simulink library "aero_libdap"  (Simulink 6.0)
settings: Solver=ode45  SolverMode=SingleTasking  StartTime=0.0  StopTime=10.0  RelTol=1e-3
values from neighbouring files (symbols this model uses):
  DB = u(6)    [aero_phaseplane.m]
  delt = 0.1    [aero_pointer_tracker.m]
undefined symbols (not defined in the file or in its folder): tmin
settings Model: CovMetricSettings=d  Creator=The MathWorks Inc.  LastModifiedBy=batserve  ExtModeAutoUpdateStatusClock=off
settings OptimizationCC: BooleanDataType=off
settings DebuggingCC: CheckExecutionContextPreStartOutputMsg=on  CheckExecutionContextRuntimeOutputMsg=on  SolverPrmCheckMsg=none
settings HardwareCC: TargetUnknown=on

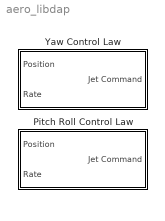
== system aero_libdap ==
  Pitch Roll Control Law : Subsystem  PropExecContextAcrossSSBoundary=on  mask(Control Law){alph=, alphs=, DB=DB, tmin=tmin, delt=delt}
      mask prompts: alph "Single Jet Accel:"; alphs "Single Jet Switch Curve Accel:"; DB "Dead Band:"; tmin "Min. Jet On Time:"; delt "Sample Time:"
      mask help: Implements Control Law for the LM. Works for yaw, u and v jet axes.
  Yaw Control Law : Subsystem  PropExecContextAcrossSSBoundary=on  mask(Control Law){alph=, alphs=, DB=DB, tmin=tmin, delt=delt}
      mask prompts: alph "Single Jet Accel:"; alphs "Single Jet Switch Curve Accel:"; DB "Dead Band:"; tmin "Min Jet On Time:"; delt "Sample Time:"
      mask help: Implements Control Law for the LM. Works for yaw, u and v jet axes.

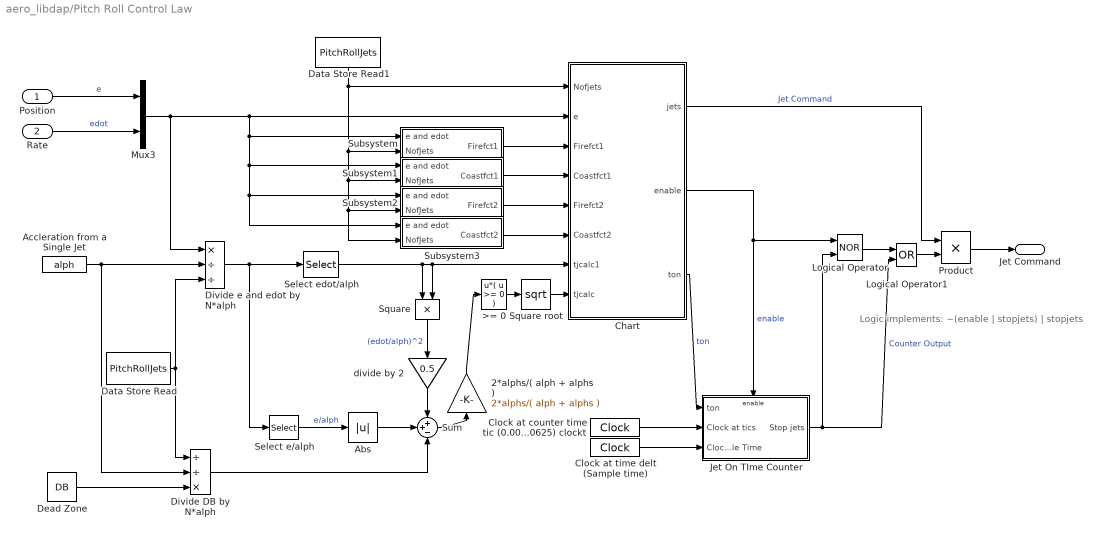
== system aero_libdap/Pitch Roll Control Law ==
  note: Logic implements:
      | ~(enable | stopjets) | stopjets
  Position : Inport  Port=1  LatchInput=off
  Rate : Inport  Port=2  LatchInput=off
  2*alphs/( alph + alphs ) : Gain  Orientation=up  Gain=2*alphs/( alph + alphs )  SaturateOnIntegerOverflow=on
  >= 0 : Fcn  Expr=u*( u >= 0 )
  Abs : Abs  SaturateOnIntegerOverflow=on
  Accleration from a Single Jet : Constant  Value=alph
  Chart : Stateflow chart  PropExecContextAcrossSSBoundary=on
  Clock at counter time tic (0.000625) clockt : DigitalClock  SampleTime=0.000625
  Clock at time delt (Sample time) : DigitalClock  SampleTime=delt
  Data Store Read : DataStoreRead  DialogController=Simulink.DDGSource  DataStoreName=PitchRollJets  SampleTime=delt
  Data Store Read1 : DataStoreRead  Orientation=down  DialogController=Simulink.DDGSource  DataStoreName=PitchRollJets  SampleTime=delt
  Dead Zone : Constant  Value=DB
  Divide e and edot by N*alph : Product  Inputs=*//  SaturateOnIntegerOverflow=on  RndMeth=Zero  InputSameDT=on
  Divide DB by N*alph : Product  Inputs=//*  SaturateOnIntegerOverflow=on  RndMeth=Zero  InputSameDT=on
  Jet On TIme Counter : Subsystem  TreatAsAtomicUnit=on  PropExecContextAcrossSSBoundary=on
  Logical Operator : Logic  Operator=NOR
  Logical Operator1 : Logic  Operator=OR
  Mux3 : Mux  Inputs=2
  Product : Product  SaturateOnIntegerOverflow=on  RndMeth=Zero  InputSameDT=on
  Select e/alph : Selector  Elements=[1]  InputPortWidth=2
  Select edot/alph : Selector  Elements=[2]  InputPortWidth=2
  Square : Product  Orientation=down  SaturateOnIntegerOverflow=on  RndMeth=Zero  InputSameDT=on
  Square root : Math  Operator=sqrt  SaturateOnIntegerOverflow=on
  Subsystem : Subsystem  PropExecContextAcrossSSBoundary=on
  Subsystem1 : Subsystem  PropExecContextAcrossSSBoundary=on
  Subsystem2 : Subsystem  PropExecContextAcrossSSBoundary=on
  Subsystem3 : Subsystem  PropExecContextAcrossSSBoundary=on
  Sum : Sum  Inputs=++-  SaturateOnIntegerOverflow=on  InputSameDT=on
  divide by 2 : Gain  Orientation=down  Gain=0.5  SaturateOnIntegerOverflow=on
  Jet Command : Outport  InitialOutput=0
  wires:
  Data Store Read1/1 -> Subsystem3/2(NofJets), Subsystem2/2(NofJets), Subsystem1/2(NofJets), Subsystem/2(NofJets), Chart/1(Nofjets)
  Rate/1 -> Mux3/2  "edot"
  Position/1 -> Mux3/1  "e"
  Mux3/1 -> Chart/2(e), Divide e and edot by N*alph/1, Subsystem/1(e and edot), Subsystem1/1(e and edot), Subsystem2/1(e and edot), Subsystem3/1(e and edot)
  Square/1 -> divide by 2/1  "(edot/alph)^2"
  Square root/1 -> Chart/8(tjcalc)
  Chart/1(jets) -> Product/1  "Jet Command"
  Select edot/alph/1 -> Square/1, Chart/7(tjcalc1), Square/2
  Select e/alph/1 -> Abs/1  "e/alph"
  divide by 2/1 -> Sum/1
  Sum/1 -> 2*alphs/( alph + alphs )/1
  Abs/1 -> Sum/2
  Divide e and edot by N*alph/1 -> Select edot/alph/1, Select e/alph/1
  Data Store Read/1 -> Divide e and edot by N*alph/3, Divide DB by N*alph/1
  Accleration from a Single Jet/1 -> Divide e and edot by N*alph/2, Divide DB by N*alph/2
  Dead Zone/1 -> Divide DB by N*alph/3
  Divide DB by N*alph/1 -> Sum/3
  Chart/2(enable) -> Jet On TIme Counter/Enable, Logical Operator/1  "enable"
  Logical Operator1/1 -> Product/2
  Chart/3(ton) -> Jet On TIme Counter/1(ton)  "ton"
  Clock at counter time tic (0.000625) clockt/1 -> Jet On TIme Counter/2(Clock at tics)
  Clock at time delt (Sample time)/1 -> Jet On TIme Counter/3(Clock at Sample Time)
  Jet On TIme Counter/1(Stop jets) -> Logical Operator/2, Logical Operator1/2  "Counter Output"
  Logical Operator/1 -> Logical Operator1/1
  Subsystem3/1(Coastfct2) -> Chart/6(Coastfct2)
  Subsystem2/1(Firefct2) -> Chart/5(Firefct2)
  Subsystem1/1(Coastfct1) -> Chart/4(Coastfct1)
  Subsystem/1(Firefct1) -> Chart/3(Firefct1)
  Product/1 -> Jet Command/1
  2*alphs/( alph + alphs )/1 -> >= 0/1
  >= 0/1 -> Square root/1

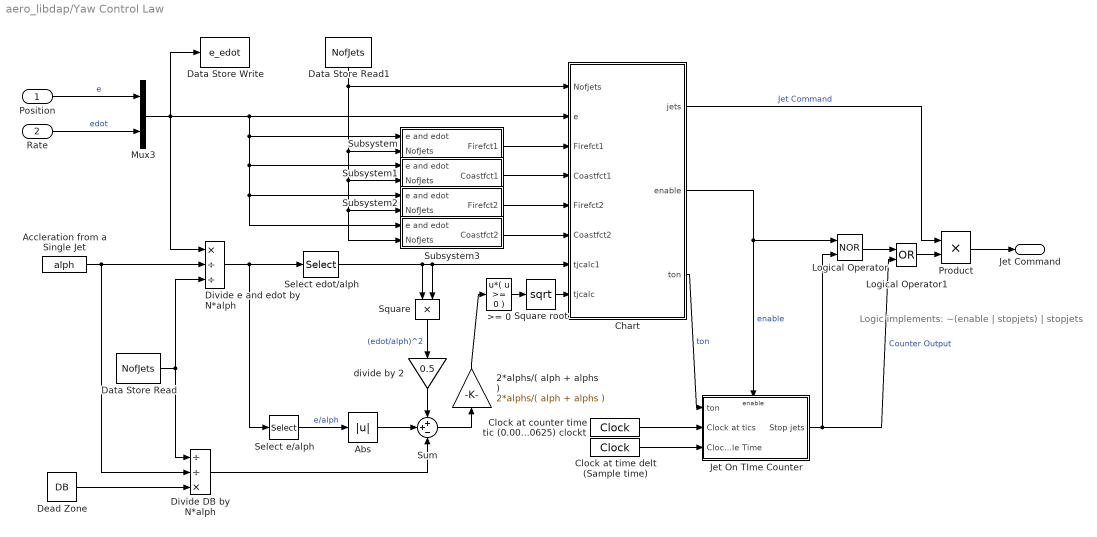
== system aero_libdap/Yaw Control Law ==
  note: Logic implements:
      | ~(enable | stopjets) | stopjets
  Position : Inport  Port=1  LatchInput=off
  Rate : Inport  Port=2  LatchInput=off
  2*alphs/( alph + alphs ) : Gain  Orientation=up  Gain=2*alphs/( alph + alphs )  SaturateOnIntegerOverflow=on
  >= 0 : Fcn  Expr=u*( u >= 0 )
  Abs : Abs  SaturateOnIntegerOverflow=on
  Accleration from a Single Jet : Constant  Value=alph
  Chart : Stateflow chart  PropExecContextAcrossSSBoundary=on
  Clock at counter time tic (0.000625) clockt : DigitalClock  SampleTime=0.000625
  Clock at time delt (Sample time) : DigitalClock  SampleTime=delt
  Data Store Read : DataStoreRead  DialogController=Simulink.DDGSource  DataStoreName=NofJets  SampleTime=delt
  Data Store Read1 : DataStoreRead  Orientation=down  DialogController=Simulink.DDGSource  DataStoreName=NofJets  SampleTime=delt
  Data Store Write : DataStoreWrite  DialogController=Simulink.DDGSource  DataStoreName=e_edot  SampleTime=-1
  Dead Zone : Constant  Value=DB
  Divide e and edot by N*alph : Product  Inputs=*//  SaturateOnIntegerOverflow=on  RndMeth=Zero  InputSameDT=on
  Divide DB by N*alph : Product  Inputs=//*  SaturateOnIntegerOverflow=on  RndMeth=Zero  InputSameDT=on
  Jet On TIme Counter : Subsystem  TreatAsAtomicUnit=on  PropExecContextAcrossSSBoundary=on
  Logical Operator : Logic  Operator=NOR
  Logical Operator1 : Logic  Operator=OR
  Mux3 : Mux  Inputs=2
  Product : Product  SaturateOnIntegerOverflow=on  RndMeth=Zero  InputSameDT=on
  Select e/alph : Selector  Elements=[1]  InputPortWidth=2
  Select edot/alph : Selector  Elements=[2]  InputPortWidth=2
  Square : Product  Orientation=down  SaturateOnIntegerOverflow=on  RndMeth=Zero  InputSameDT=on
  Square root : Math  Operator=sqrt  SaturateOnIntegerOverflow=on
  Subsystem : Subsystem  PropExecContextAcrossSSBoundary=on
  Subsystem1 : Subsystem  PropExecContextAcrossSSBoundary=on
  Subsystem2 : Subsystem  PropExecContextAcrossSSBoundary=on
  Subsystem3 : Subsystem  PropExecContextAcrossSSBoundary=on
  Sum : Sum  Inputs=++-  SaturateOnIntegerOverflow=on  InputSameDT=on
  divide by 2 : Gain  Orientation=down  Gain=0.5  SaturateOnIntegerOverflow=on
  Jet Command : Outport  InitialOutput=0
  wires:
  Product/1 -> Jet Command/1
  Subsystem/1(Firefct1) -> Chart/3(Firefct1)
  Subsystem1/1(Coastfct1) -> Chart/4(Coastfct1)
  Subsystem2/1(Firefct2) -> Chart/5(Firefct2)
  Subsystem3/1(Coastfct2) -> Chart/6(Coastfct2)
  Logical Operator/1 -> Logical Operator1/1
  Jet On TIme Counter/1(Stop jets) -> Logical Operator1/2, Logical Operator/2  "Counter Output"
  Clock at time delt (Sample time)/1 -> Jet On TIme Counter/3(Clock at Sample Time)
  Clock at counter time tic (0.000625) clockt/1 -> Jet On TIme Counter/2(Clock at tics)
  Chart/3(ton) -> Jet On TIme Counter/1(ton)  "ton"
  Logical Operator1/1 -> Product/2
  Chart/2(enable) -> Logical Operator/1, Jet On TIme Counter/Enable  "enable"
  Divide DB by N*alph/1 -> Sum/3
  Dead Zone/1 -> Divide DB by N*alph/3
  Accleration from a Single Jet/1 -> Divide DB by N*alph/2, Divide e and edot by N*alph/2
  Data Store Read/1 -> Divide DB by N*alph/1, Divide e and edot by N*alph/3
  Divide e and edot by N*alph/1 -> Select e/alph/1, Select edot/alph/1
  Abs/1 -> Sum/2
  Sum/1 -> 2*alphs/( alph + alphs )/1
  divide by 2/1 -> Sum/1
  Select e/alph/1 -> Abs/1  "e/alph"
  Select edot/alph/1 -> Square/2, Chart/7(tjcalc1), Square/1
  Chart/1(jets) -> Product/1  "Jet Command"
  Square root/1 -> Chart/8(tjcalc)
  Square/1 -> divide by 2/1  "(edot/alph)^2"
  Mux3/1 -> Subsystem3/1(e and edot), Subsystem2/1(e and edot), Subsystem1/1(e and edot), Subsystem/1(e and edot), Divide e and edot by N*alph/1, Chart/2(e), Data Store Write/1
  Position/1 -> Mux3/1  "e"
  Rate/1 -> Mux3/2  "edot"
  Data Store Read1/1 -> Chart/1(Nofjets), Subsystem/2(NofJets), Subsystem1/2(NofJets), Subsystem2/2(NofJets), Subsystem3/2(NofJets)
  2*alphs/( alph + alphs )/1 -> >= 0/1
  >= 0/1 -> Square root/1

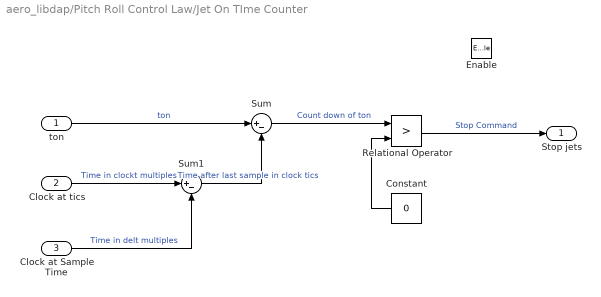
== system aero_libdap/Pitch Roll Control Law/Jet On TIme Counter ==
  ton : Inport  Port=1  LatchInput=off
  Clock at tics : Inport  Port=2  LatchInput=off
  Clock at Sample Time : Inport  Port=3  LatchInput=off
  Enable : EnablePort  StatesWhenEnabling=reset
  Constant : Constant  Orientation=left  Value=0
  Relational Operator : RelationalOperator  Operator=>  InputSameDT=on
  Sum : Sum  Inputs=|+-  SaturateOnIntegerOverflow=on  InputSameDT=on
  Sum1 : Sum  Inputs=|+-  SaturateOnIntegerOverflow=on  InputSameDT=on
  Stop jets : Outport
  wires:
  Constant/1 -> Relational Operator/2
  ton/1 -> Sum/1  "ton"
  Clock at tics/1 -> Sum1/1  "Time in clockt multiples"
  Clock at Sample Time/1 -> Sum1/2  "Time in delt multiples"
  Sum1/1 -> Sum/2  "Time after last sample in clock tics"
  Sum/1 -> Relational Operator/1  "Count down of ton"
  Relational Operator/1 -> Stop jets/1  "Stop Command"

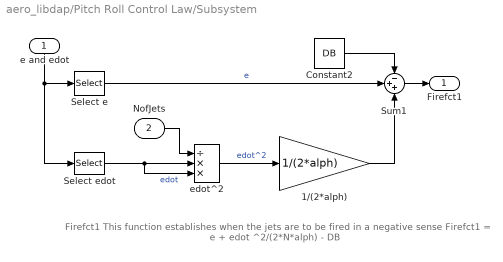
== system aero_libdap/Pitch Roll Control Law/Subsystem ==
  note: Firefct1
      | This function establishes when the jets are to be fired in a negative sense
      | Firefct1 = e + edot ^2/(2*N*alph) - DB
  e and edot : Inport  Orientation=down  Port=1  LatchInput=off
  NofJets : Inport  Port=2  LatchInput=off
  1/(2*alph) : Gain  Gain=1/(2*alph)  SaturateOnIntegerOverflow=on
  Constant2 : Constant  Value=DB
  Select e : Selector  Elements=[1]  InputPortWidth=2
  Select edot : Selector  Elements=[2]  InputPortWidth=2
  Sum1 : Sum  Inputs=-++  SaturateOnIntegerOverflow=on  InputSameDT=on
  edot^2 : Product  Inputs=/**  SaturateOnIntegerOverflow=on  RndMeth=Zero  InputSameDT=on
  Firefct1 : Outport
  wires:
  edot^2/1 -> 1/(2*alph)/1  "edot^2"
  Select edot/1 -> edot^2/2, edot^2/3  "edot"
  NofJets/1 -> edot^2/1
  e and edot/1 -> Select e/1, Select edot/1
  1/(2*alph)/1 -> Sum1/3
  Constant2/1 -> Sum1/1
  Select e/1 -> Sum1/2  "e"
  Sum1/1 -> Firefct1/1

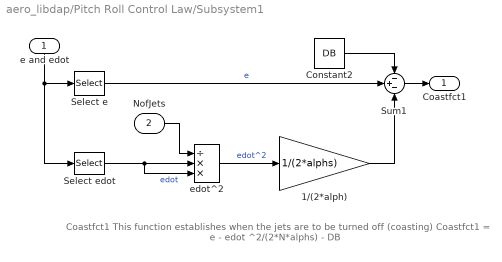
== system aero_libdap/Pitch Roll Control Law/Subsystem1 ==
  note: Coastfct1
      | This function establishes when the jets are to be turned off (coasting)
      | Coastfct1 = e - edot ^2/(2*N*alphs) - DB
  e and edot : Inport  Orientation=down  Port=1  LatchInput=off
  NofJets : Inport  Port=2  LatchInput=off
  1/(2*alph) : Gain  Gain=1/(2*alphs)  SaturateOnIntegerOverflow=on
  Constant2 : Constant  Value=DB
  Select e : Selector  Elements=[1]  InputPortWidth=2
  Select edot : Selector  Elements=[2]  InputPortWidth=2
  Sum1 : Sum  Inputs=-+-  SaturateOnIntegerOverflow=on  InputSameDT=on
  edot^2 : Product  Inputs=/**  SaturateOnIntegerOverflow=on  RndMeth=Zero  InputSameDT=on
  Coastfct1 : Outport
  wires:
  Sum1/1 -> Coastfct1/1
  Select e/1 -> Sum1/2  "e"
  Constant2/1 -> Sum1/1
  1/(2*alph)/1 -> Sum1/3
  e and edot/1 -> Select edot/1, Select e/1
  NofJets/1 -> edot^2/1
  Select edot/1 -> edot^2/3, edot^2/2  "edot"
  edot^2/1 -> 1/(2*alph)/1  "edot^2"

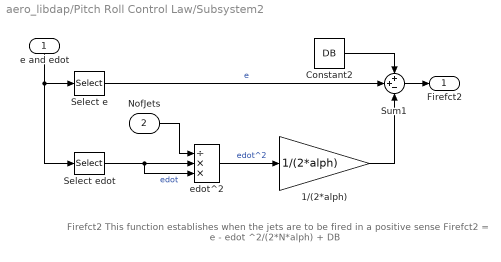
== system aero_libdap/Pitch Roll Control Law/Subsystem2 ==
  note: Firefct2
      | This function establishes when the jets are to be fired in a positive sense
      | Firefct2 = e - edot ^2/(2*N*alph) + DB
  e and edot : Inport  Orientation=down  Port=1  LatchInput=off
  NofJets : Inport  Port=2  LatchInput=off
  1/(2*alph) : Gain  Gain=1/(2*alph)  SaturateOnIntegerOverflow=on
  Constant2 : Constant  Value=DB
  Select e : Selector  Elements=[1]  InputPortWidth=2
  Select edot : Selector  Elements=[2]  InputPortWidth=2
  Sum1 : Sum  Inputs=++-  SaturateOnIntegerOverflow=on  InputSameDT=on
  edot^2 : Product  Inputs=/**  SaturateOnIntegerOverflow=on  RndMeth=Zero  InputSameDT=on
  Firefct2 : Outport
  wires:
  edot^2/1 -> 1/(2*alph)/1  "edot^2"
  Select edot/1 -> edot^2/2, edot^2/3  "edot"
  NofJets/1 -> edot^2/1
  e and edot/1 -> Select e/1, Select edot/1
  1/(2*alph)/1 -> Sum1/3
  Constant2/1 -> Sum1/1
  Select e/1 -> Sum1/2  "e"
  Sum1/1 -> Firefct2/1

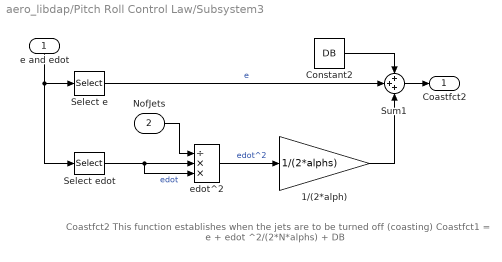
== system aero_libdap/Pitch Roll Control Law/Subsystem3 ==
  note: Coastfct2
      | This function establishes when the jets are to be turned off (coasting)
      | Coastfct1 = e + edot ^2/(2*N*alphs) + DB
  e and edot : Inport  Orientation=down  Port=1  LatchInput=off
  NofJets : Inport  Port=2  LatchInput=off
  1/(2*alph) : Gain  Gain=1/(2*alphs)  SaturateOnIntegerOverflow=on
  Constant2 : Constant  Value=DB
  Select e : Selector  Elements=[1]  InputPortWidth=2
  Select edot : Selector  Elements=[2]  InputPortWidth=2
  Sum1 : Sum  Inputs=+++  SaturateOnIntegerOverflow=on  InputSameDT=on
  edot^2 : Product  Inputs=/**  SaturateOnIntegerOverflow=on  RndMeth=Zero  InputSameDT=on
  Coastfct2 : Outport
  wires:
  edot^2/1 -> 1/(2*alph)/1  "edot^2"
  Select edot/1 -> edot^2/2, edot^2/3  "edot"
  NofJets/1 -> edot^2/1
  e and edot/1 -> Select e/1, Select edot/1
  1/(2*alph)/1 -> Sum1/3
  Constant2/1 -> Sum1/1
  Select e/1 -> Sum1/2  "e"
  Sum1/1 -> Coastfct2/1

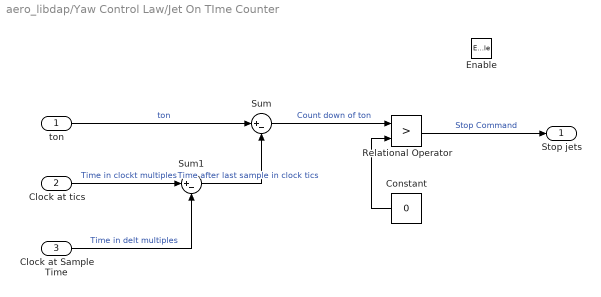
== system aero_libdap/Yaw Control Law/Jet On TIme Counter ==
  ton : Inport  Port=1  LatchInput=off
  Clock at tics : Inport  Port=2  LatchInput=off
  Clock at Sample Time : Inport  Port=3  LatchInput=off
  Enable : EnablePort  StatesWhenEnabling=reset
  Constant : Constant  Orientation=left  Value=0
  Relational Operator : RelationalOperator  Operator=>  InputSameDT=on
  Sum : Sum  Inputs=|+-  SaturateOnIntegerOverflow=on  InputSameDT=on
  Sum1 : Sum  Inputs=|+-  SaturateOnIntegerOverflow=on  InputSameDT=on
  Stop jets : Outport
  wires:
  Relational Operator/1 -> Stop jets/1  "Stop Command"
  Sum/1 -> Relational Operator/1  "Count down of ton"
  Sum1/1 -> Sum/2  "Time after last sample in clock tics"
  Clock at Sample Time/1 -> Sum1/2  "Time in delt multiples"
  Clock at tics/1 -> Sum1/1  "Time in clockt multiples"
  ton/1 -> Sum/1  "ton"
  Constant/1 -> Relational Operator/2

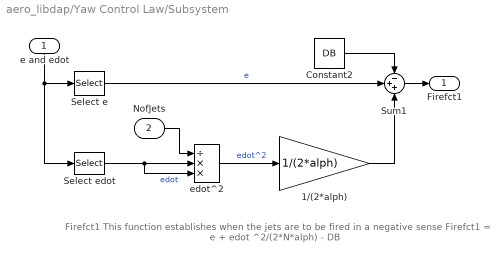
== system aero_libdap/Yaw Control Law/Subsystem ==
  note: Firefct1
      | This function establishes when the jets are to be fired in a negative sense
      | Firefct1 = e + edot ^2/(2*N*alph) - DB
  e and edot : Inport  Orientation=down  Port=1  LatchInput=off
  NofJets : Inport  Port=2  LatchInput=off
  1/(2*alph) : Gain  Gain=1/(2*alph)  SaturateOnIntegerOverflow=on
  Constant2 : Constant  Value=DB
  Select e : Selector  Elements=[1]  InputPortWidth=2
  Select edot : Selector  Elements=[2]  InputPortWidth=2
  Sum1 : Sum  Inputs=-++  SaturateOnIntegerOverflow=on  InputSameDT=on
  edot^2 : Product  Inputs=/**  SaturateOnIntegerOverflow=on  RndMeth=Zero  InputSameDT=on
  Firefct1 : Outport
  wires:
  Sum1/1 -> Firefct1/1
  Select e/1 -> Sum1/2  "e"
  Constant2/1 -> Sum1/1
  1/(2*alph)/1 -> Sum1/3
  e and edot/1 -> Select edot/1, Select e/1
  NofJets/1 -> edot^2/1
  Select edot/1 -> edot^2/3, edot^2/2  "edot"
  edot^2/1 -> 1/(2*alph)/1  "edot^2"

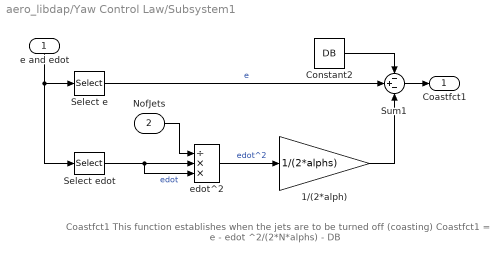
== system aero_libdap/Yaw Control Law/Subsystem1 ==
  note: Coastfct1
      | This function establishes when the jets are to be turned off (coasting)
      | Coastfct1 = e - edot ^2/(2*N*alphs) - DB
  e and edot : Inport  Orientation=down  Port=1  LatchInput=off
  NofJets : Inport  Port=2  LatchInput=off
  1/(2*alph) : Gain  Gain=1/(2*alphs)  SaturateOnIntegerOverflow=on
  Constant2 : Constant  Value=DB
  Select e : Selector  Elements=[1]  InputPortWidth=2
  Select edot : Selector  Elements=[2]  InputPortWidth=2
  Sum1 : Sum  Inputs=-+-  SaturateOnIntegerOverflow=on  InputSameDT=on
  edot^2 : Product  Inputs=/**  SaturateOnIntegerOverflow=on  RndMeth=Zero  InputSameDT=on
  Coastfct1 : Outport
  wires:
  edot^2/1 -> 1/(2*alph)/1  "edot^2"
  Select edot/1 -> edot^2/2, edot^2/3  "edot"
  NofJets/1 -> edot^2/1
  e and edot/1 -> Select e/1, Select edot/1
  1/(2*alph)/1 -> Sum1/3
  Constant2/1 -> Sum1/1
  Select e/1 -> Sum1/2  "e"
  Sum1/1 -> Coastfct1/1

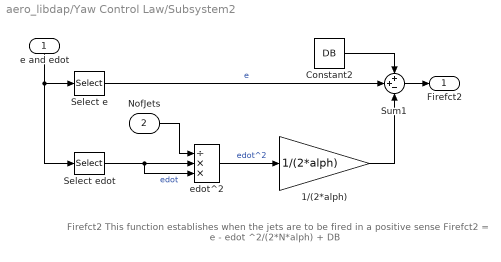
== system aero_libdap/Yaw Control Law/Subsystem2 ==
  note: Firefct2
      | This function establishes when the jets are to be fired in a positive sense
      | Firefct2 = e - edot ^2/(2*N*alph) + DB
  e and edot : Inport  Orientation=down  Port=1  LatchInput=off
  NofJets : Inport  Port=2  LatchInput=off
  1/(2*alph) : Gain  Gain=1/(2*alph)  SaturateOnIntegerOverflow=on
  Constant2 : Constant  Value=DB
  Select e : Selector  Elements=[1]  InputPortWidth=2
  Select edot : Selector  Elements=[2]  InputPortWidth=2
  Sum1 : Sum  Inputs=++-  SaturateOnIntegerOverflow=on  InputSameDT=on
  edot^2 : Product  Inputs=/**  SaturateOnIntegerOverflow=on  RndMeth=Zero  InputSameDT=on
  Firefct2 : Outport
  wires:
  Sum1/1 -> Firefct2/1
  Select e/1 -> Sum1/2  "e"
  Constant2/1 -> Sum1/1
  1/(2*alph)/1 -> Sum1/3
  e and edot/1 -> Select edot/1, Select e/1
  NofJets/1 -> edot^2/1
  Select edot/1 -> edot^2/3, edot^2/2  "edot"
  edot^2/1 -> 1/(2*alph)/1  "edot^2"

== system aero_libdap/Yaw Control Law/Subsystem3 ==
  note: Coastfct2
      | This function establishes when the jets are to be turned off (coasting)
      | Coastfct1 = e + edot ^2/(2*N*alphs) + DB
  e and edot : Inport  Orientation=down  Port=1  LatchInput=off
  NofJets : Inport  Port=2  LatchInput=off
  1/(2*alph) : Gain  Gain=1/(2*alphs)  SaturateOnIntegerOverflow=on
  Constant2 : Constant  Value=DB
  Select e : Selector  Elements=[1]  InputPortWidth=2
  Select edot : Selector  Elements=[2]  InputPortWidth=2
  Sum1 : Sum  Inputs=+++  SaturateOnIntegerOverflow=on  InputSameDT=on
  edot^2 : Product  Inputs=/**  SaturateOnIntegerOverflow=on  RndMeth=Zero  InputSameDT=on
  Coastfct2 : Outport
  wires:
  Sum1/1 -> Coastfct2/1
  Select e/1 -> Sum1/2  "e"
  Constant2/1 -> Sum1/1
  1/(2*alph)/1 -> Sum1/3
  e and edot/1 -> Select edot/1, Select e/1
  NofJets/1 -> edot^2/1
  Select edot/1 -> edot^2/3, edot^2/2  "edot"
  edot^2/1 -> 1/(2*alph)/1  "edot^2"

== stateflow chart Pitch Roll Control Law/Chart ==
  settings: updateMethod=DISCRETE  sampleTime=delt
  state Wait_for_stable_rate
  state Start
  state Fire_region_1
    en: jets=-Nofjets;
    ton=tjcalc+tjcalc1;
  state Coast_region_2
    en: jets=0;
    ton=0;
    enable=0;
  state Skip_a_Sample_2
    en:count--;
  state Skip_a_Sample_1
    en:count--;
  state Coast_region_1
    en: jets=0;
    ton=0;
    enable=0;
  state Fire_region_2
    en: jets=Nofjets;
    ton=tjcalc-tjcalc1;
  Wait_for_stable_rate -> Start : [count==0]
  (default) -> Wait_for_stable_rate : /count=2;
  Wait_for_stable_rate -> Wait_for_stable_rate : /count--;
  Start -> Fire_region_2 : [ (e[1]<0 & Firefct2<0) | (e[1]>0 & Coastfct2>0) ]
  Start -> Coast_region_1 : [ (e[1]<0 & Coastfct1<=0 & Firefct2>0) ]
  Start -> Coast_region_2 : [ (e[1]>0 & Coastfct2>=0 & Firefct1<0) ]
  Start -> Fire_region_1 : [ (e[1]>0 & Firefct1>0) | (e[1]<0 & Coastfct1<0) ]
  Coast_region_2 -> Fire_region_1 : [e[1]>0 & Firefct1>0]
  Skip_a_Sample_2 -> Coast_region_2 : [count==0]
  Fire_region_1 -> Fire_region_1
  Fire_region_1 -> (junction 11) : [ton<2*delt]{enable=1;}
  Fire_region_1 -> Coast_region_1 : [e[1]<0 & Coastfct1<=0]
  (junction 12) -> Coast_region_2 : {enable=0;}
  Fire_region_2 -> Coast_region_2 : [e[1]>0 & Coastfct2>0]
  (junction 11) -> Coast_region_1 : {enable=0;}
  Skip_a_Sample_2 -> Skip_a_Sample_2 : /ton=ton-delt;
  (junction 11) -> Skip_a_Sample_1 : [ton>tmin]{count=2;}
  (junction 12) -> Skip_a_Sample_2 : [ton>tmin]{count=2;}
  Skip_a_Sample_1 -> Skip_a_Sample_1 : /ton=ton-delt;
  Skip_a_Sample_1 -> Coast_region_1 : [count==0]
  Fire_region_2 -> (junction 12) : [ton<2*delt]{enable=1;}
  Coast_region_1 -> Fire_region_2 : [e[1]<0 & Firefct2<0]
  Fire_region_2 -> Fire_region_2
  data: jets output double; Nofjets input double; e input double size=2; enable output double; ton output double; Firefct1 input double; Coastfct1 input double; Firefct2 input double; Coastfct2 input double; tjcalc1 input double; tjcalc input double; tmin parameter double; delt parameter double; count local double

== stateflow chart Yaw Control Law/Chart ==
  settings: updateMethod=DISCRETE  sampleTime=delt
  state Wait_for_stable_rate
  state Start
  state Fire_region_1
    en: jets=-Nofjets;
    ton=tjcalc+tjcalc1;
  state Coast_region_2
    en: jets=0;
    ton=0;
    enable=0;
  state Skip_a_Sample_2
    en:count--;
  state Skip_a_Sample_1
    en:count--;
  state Coast_region_1
    en: jets=0;
    ton=0;
    enable=0;
  state Fire_region_2
    en: jets=Nofjets;
    ton=tjcalc-tjcalc1;
  Wait_for_stable_rate -> Start : [count==0]
  (default) -> Wait_for_stable_rate : /count=2;
  Wait_for_stable_rate -> Wait_for_stable_rate : /count--;
  Start -> Fire_region_2 : [ (e[1]<0 & Firefct2<0) | (e[1]>0 & Coastfct2>0) ]
  Start -> Coast_region_1 : [ (e[1]<0 & Coastfct1<=0 & Firefct2>0) ]
  Start -> Coast_region_2 : [ (e[1]>0 & Coastfct2>=0 & Firefct1<0) ]
  Start -> Fire_region_1 : [ (e[1]>0 & Firefct1>0) | (e[1]<0 & Coastfct1<0) ]
  Coast_region_2 -> Fire_region_1 : [e[1]>0 & Firefct1>0]
  Skip_a_Sample_2 -> Coast_region_2 : [count==0]
  Fire_region_1 -> Fire_region_1
  Fire_region_1 -> (junction 60) : [ton<2*delt]{enable=1;}
  Fire_region_1 -> Coast_region_1 : [e[1]<0 & Coastfct1<=0]
  (junction 61) -> Coast_region_2 : {enable=0;}
  Fire_region_2 -> Coast_region_2 : [e[1]>0 & Coastfct2>0]
  (junction 60) -> Coast_region_1 : {enable=0;}
  Skip_a_Sample_2 -> Skip_a_Sample_2 : /ton=ton-delt;
  (junction 60) -> Skip_a_Sample_1 : [ton>tmin]{count=2;}
  (junction 61) -> Skip_a_Sample_2 : [ton>tmin]{count=2;}
  Skip_a_Sample_1 -> Skip_a_Sample_1 : /ton=ton-delt;
  Skip_a_Sample_1 -> Coast_region_1 : [count==0]
  Fire_region_2 -> (junction 61) : [ton<2*delt]{enable=1;}
  Coast_region_1 -> Fire_region_2 : [e[1]<0 & Firefct2<0]
  Fire_region_2 -> Fire_region_2
  data: jets output double; Nofjets input double; e input double size=2; enable output double; ton output double; Firefct1 input double; Coastfct1 input double; Firefct2 input double; Coastfct2 input double; tjcalc1 input double; tjcalc input double; tmin parameter double; delt parameter double; count local double
